simulink model "Prob_1c_d"  (R2016b)
settings: Solver=VariableStepAuto  StartTime=0.0  StopTime=10.0  RelTol=1e-3
values from neighbouring files (symbols this model uses):
  A = []    [Parameters_1c_d.m]
  B = []    [Parameters_1c_d.m]
  C = [1 0 0 --- 1]    [Parameters_1c_d.m]
  D = 0    [Parameters_1c_d.m]
settings Model: Creator=helene  LastModifiedBy=helene

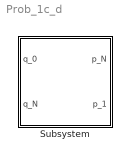
== system Prob_1c_d ==
  Subsystem : Subsystem

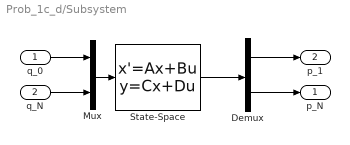
== system Prob_1c_d/Subsystem ==
  q_0 : Inport
  q_N : Inport  Port=2
  Demux : Demux  Outputs=2
  Mux : Mux  Inputs=2
  State-Space : StateSpace  A=A  B=B  C=C  D=D  X0=0
  p_N : Outport
  p_1 : Outport  Port=2
  wires:
  Mux/1 -> State-Space/1
  q_N/1 -> Mux/2
  q_0/1 -> Mux/1
  State-Space/1 -> Demux/1
  Demux/2 -> p_N/1
  Demux/1 -> p_1/1
